simulink model "ProbeModel_Pseudo"  (R2025a)
settings: Solver=ode23tb  StartTime=0.0  StopTime=1000  MaxStep=0.1  RelTol=1e-3
model workspace (MAT data in the model file):
  pseudo_dx = 55
  pseudo_dy = 0
  tank_height = 22
  tank_wl_min = 83
settings Model: DataDictionary=FuelGaugingData.sldd  Creator=mkelley  LastModifiedBy=mkelley

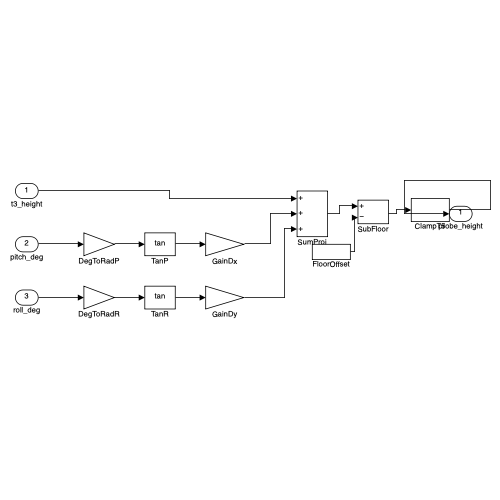
[thumbnail: Simulink's stored preview of the top-level diagram]
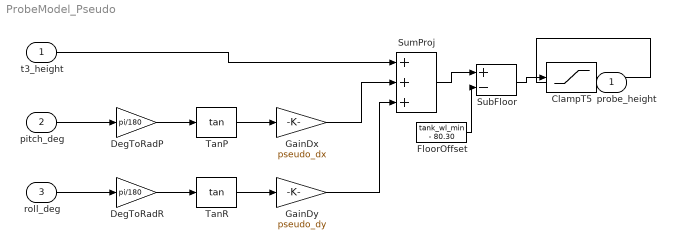
== system ProbeModel_Pseudo ==
  t3_height : Inport
  pitch_deg : Inport  Port=2
  roll_deg : Inport  Port=3
  ClampT5 : Saturate  UpperLimit=tank_height  LowerLimit=0
  DegToRadP : Gain  Gain=pi/180
  DegToRadR : Gain  Gain=pi/180
  FloorOffset : Constant  Value=tank_wl_min - 80.30
  GainDx : Gain  Gain=pseudo_dx
  GainDy : Gain  Gain=pseudo_dy
  SubFloor : Sum  Inputs=+-
  SumProj : Sum  Inputs=+++
  TanP : Trigonometry  Operator=tan
  TanR : Trigonometry  Operator=tan
  probe_height : Outport
  wires:
  pitch_deg/1 -> DegToRadP/1
  DegToRadP/1 -> TanP/1
  TanP/1 -> GainDx/1
  roll_deg/1 -> DegToRadR/1
  DegToRadR/1 -> TanR/1
  TanR/1 -> GainDy/1
  t3_height/1 -> SumProj/1
  GainDx/1 -> SumProj/2
  GainDy/1 -> SumProj/3
  SumProj/1 -> SubFloor/1
  FloorOffset/1 -> SubFloor/2
  SubFloor/1 -> ClampT5/1
  ClampT5/1 -> probe_height/1
